simulink model "Processo"  (R2021b)
settings: Solver=ode4  StartTime=0.0  StopTime=1000  FixedStep=1e-1  RelTol=1e-3
model workspace (MAT data in the model file):
  plant_dist = [0  3  3  3  5  4  8  8  6; 3  0  3  3  5  5  8  6  4; 3  3  0  1  3  3  8  6  4; 3  3  1  0  3  3  8  6  4; 5  5  3  3  0  3  6  4  2; 4  5  3  3  3  0  6  6  4; 8  8  8  8  6  6  0  3  5; 8  6  6  6  4  6  3  0  3; 6  4  4  4  2  4  5  3  0]
undefined symbols (not defined in the file): entity, getAttribute, m, n
libraries: simulink x2, sldelib x1
settings Model: PauseTimes=0  Creator=chrez  LastModifiedBy=chrez

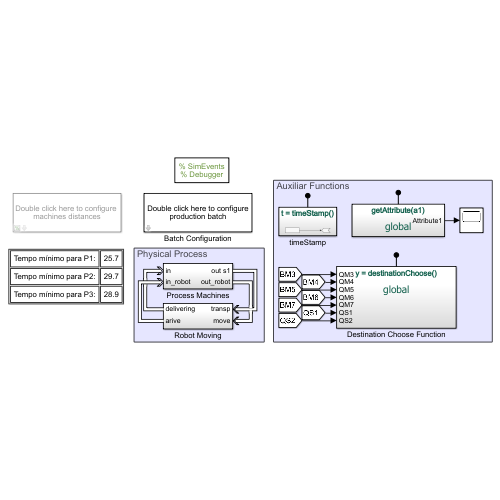
[thumbnail: Simulink's stored preview of the top-level diagram]
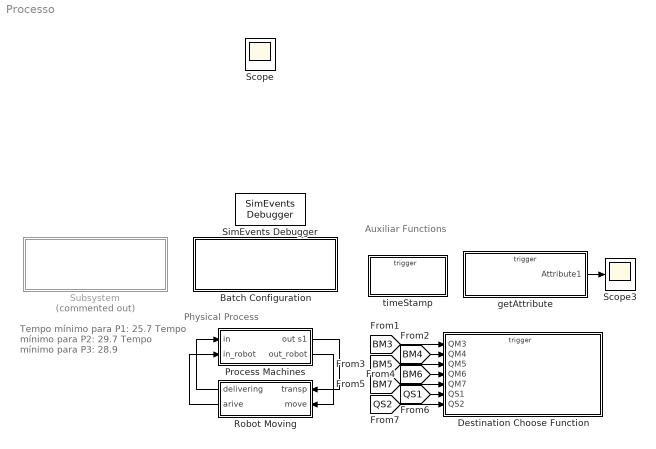
== system Processo ==
  note: Physical Process
  note: Auxiliar Functions
  note: Tempo mínimo para P1:
      | 25.7
      |
      | Tempo mínimo para P2:
      | 29.7
      |
      | Tempo mínimo para P3:
      | 28.9
  Batch Configuration : Subsystem  mask(Batch Configuration){bp1=9, bp2=5, bp3=7, t1recipe=[1 3 4 5 8], t1serviceTimes=[5 3.8 2.5 1.9 1.5], t2recipe=[1 3 6 7 8], t2serviceTimes=[5 3.2 2.4 1.6 2.5], t3recipe=[2 4 5 7 8], t3serviceTimes=[4 2.5 2.4 2.5 2.5]}
      mask prompts: bp1 "Type 1:"; bp2 "Type 2:"; bp3 "Type 3:"; t1recipe "Recipe:"; t1serviceTimes "Service Times:"; t2recipe "Recipe:"; t2serviceTimes "Service Times:"; t3recipe "Recipe:"; t3serviceTimes "Service Times:"
      mask init:
      | assignin('base','bp1',bp1);
      | assignin('base','bp2',bp2);
      | assignin('base','bp3',bp3);
      | assignin('base','t1recipe',t1recipe);
      | assignin('base','t2recipe',t2recipe);
      | assignin('base','t3recipe',t3recipe);
      | assignin('base','t1serviceTimes',t1serviceTimes);
      | assignin('base','t2serviceTimes',t2serviceTimes);
      | assignin('base','t3serviceTimes',t3serviceTimes);
      mask DialogControl ParameterGroupVar Prompt: Batch Query
      mask DialogControl Container7 Prompt: Parts Configuration
      mask DialogControl Container5 Prompt: Type 1
      mask DialogControl Container6 Prompt: Type 2
      mask DialogControl Container10 Prompt: Type 3
      mask Display: disp('Double click here to configure\nproduction batch')
  Destination Choose Function : Subsystem  TreatAsAtomicUnit=on
  Process Machines : Subsystem
  Robot Moving : Subsystem
      settings: PortSchema="{\"entries\":[{\"content\":{\"sides\":[{\"content\":{\"connectorIds\":[\"Out1\",\"Out2\"]},\"type\":\"ConnectorPlacement.EquallySpacedRectSide\",\"uuid\":\"7e07b981-1494-4663-ac57-34fb851c4f8b\"},{\"content\":{\"connectorIds\":[\"In1\",\"In2\"],\"side\":\"RIGHT\"},\"type\":\"ConnectorPlacement.EquallySpacedRectSide\",\"uuid\":\"835ab307-364b-4a91-b206-e24ceecefc82\"},{\"content\":{\"connectorIds\":[],\"side\":\"TOP\"},\"type\":\"ConnectorPlacement.EquallySpacedRectSide\",\"uuid\":\"da88ac6b-0800-49ec-b50d-c8d35a849956\"}]},\"type\":\"ConnectorPlacement.EquallySpacedConnector\",\"uuid\":\"81c2c33b-7057-4473-b38a-1a0a1e572193\"}],\"packageUris\":[\"http://schema.mathworks.com/mf0/Connector/R2020b\"],\"version\":\"1.0\"}"
  Scope3 : Scope
  SimEvents Debugger : sldelib/SimEvents Debugger  EnableDebugger=off  ShowInLibBrowser=0
      settings: SourceProductBaseCode=SE
  Subsystem : Subsystem  Commented=on  mask{m1_2=0, m1_2_copy=0, m1_2_copy_copy=0, m1_2_copy_copy_copy=0, m1_2_copy_copy_copy_copy=0, m1_2_copy_copy_copy_copy_copy=0, m1_2_copy_copy_copy_copy_copy_copy=0, m1_2_copy_copy_copy_copy_copy_copy_copy=0}
      mask prompts: m1_2 "1 - 2"; m1_2_copy "1 - 3"; m1_2_copy_copy "1 - 4"; m1_2_copy_copy_copy "1 - 5"; m1_2_copy_copy_copy_copy "1 - 6"; m1_2_copy_copy_copy_copy_copy "1 - 7"; m1_2_copy_copy_copy_copy_copy_copy "1 - 8"; m1_2_copy_copy_copy_copy_copy_copy_copy "1 - 9"
      mask DialogControl Container3 Prompt: Distances
      mask Display: disp('Double click here to configure \nmachines distances')
  getAttribute : Subsystem  TreatAsAtomicUnit=on
  timeStamp : Subsystem  TreatAsAtomicUnit=on
  Scope : Scope
  wires:
  Process Machines/1(out s1) -> Robot Moving/1(transp)
  Robot Moving/1(delivering) -> Process Machines/1(in)
  Process Machines/2(out_robot) -> Robot Moving/2(move)
  Robot Moving/2(arive) -> Process Machines/2(in_robot)
  [BM3] -> Destination Choose Function/1(QM3)
  [BM4] -> Destination Choose Function/2(QM4)
  [BM5] -> Destination Choose Function/3(QM5)
  [BM6] -> Destination Choose Function/4(QM6)
  [BM7] -> Destination Choose Function/5(QM7)
  getAttribute/1(Attribute1) -> Scope3/1
  [QS1] -> Destination Choose Function/6(QS1)
  [QS2] -> Destination Choose Function/7(QS2)

== system Processo/Batch Configuration ==

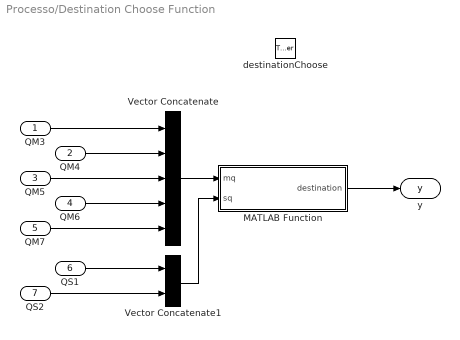
== system Processo/Destination Choose Function ==
  QM3 : Inport
  QM4 : Inport  Port=2
  QM5 : Inport  Port=3
  QM6 : Inport  Port=4
  QM7 : Inport  Port=5
  QS1 : Inport  Port=6
  QS2 : Inport  Port=7
  destinationChoose : TriggerPort  TriggerType=function-call  IsSimulinkFunction=on  FunctionName=destinationChoose  VariantControl=(inherit)
  MATLAB Function : MATLAB Function  TreatAsAtomicUnit=on
  Vector Concatenate : Concatenate  NumInputs=5
  Vector Concatenate1 : Concatenate
  y : ArgOut  DisableCoverage=on  ArgumentName=y
  wires:
  MATLAB Function/1(destination) -> y/1
  QM3/1 -> Vector Concatenate/1
  Vector Concatenate/1 -> MATLAB Function/1(mq)
  QM4/1 -> Vector Concatenate/2
  QM5/1 -> Vector Concatenate/3
  QM6/1 -> Vector Concatenate/4
  QM7/1 -> Vector Concatenate/5
  Vector Concatenate1/1 -> MATLAB Function/2(sq)
  QS2/1 -> Vector Concatenate1/2
  QS1/1 -> Vector Concatenate1/1

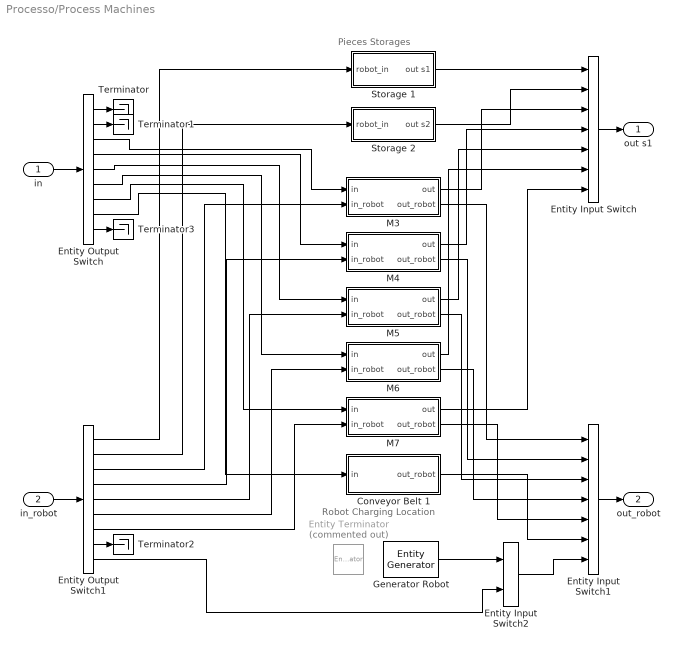
== system Processo/Process Machines ==
  note: Robot Charging Location
  note: Pieces Storages
  in : Inport
  in_robot : Inport  Port=2
  Conveyor Belt 1 : Subsystem
  Entity Input Switch : EntityInputSwitch  InputPortMessageModes=m,m,m,m,m,m,m  OutputPortMessageModes=m  NumberInputPorts=7
      settings: InputPortMap=u1,u2,u3,u4,u5,u6,u7
  Entity Input Switch1 : EntityInputSwitch  InputPortMessageModes=m,m,m,m,m,m,m  OutputPortMessageModes=m  NumberInputPorts=7
      settings: InputPortMap=u1,u2,u3,u4,u5,u6,u7
  Entity Input Switch2 : EntityInputSwitch  InputPortMessageModes=m,m  OutputPortMessageModes=m
  Entity Output Switch : EntityOutputSwitch  InputPortMessageModes=m  OutputPortMessageModes=m,m,m,m,m,m,m,m,m  NumberOutputPorts=9  SwitchingCriterion=From attribute  SwitchAttributeName=robot.atPlace
      settings: OutputPortMap=o0,o1,o2,o3,o4,o5,o6,o7,o8
  Entity Output Switch1 : EntityOutputSwitch  InputPortMessageModes=m  OutputPortMessageModes=m,m,m,m,m,m,m,m,m  NumberOutputPorts=9  SwitchingCriterion=From attribute  SwitchAttributeName=atPlace
      settings: OutputPortMap=o0,o1,o2,o3,o4,o5,o6,o7,o8
  Entity Terminator : EntityTerminator  Commented=on  InputPortMessageModes=m
  Generator Robot : EntityGenerator  OutputPortMessageModes=m  TimeSource=MATLAB action  IntergenerationTimeAction=|  GenerateEntityAtSimulationStart=off  GenerateAction=|  AttributeName=isMoving|atPlace|load|destination  AttributeInitialValue=false|9|0|0  EntityType=Structured  EntityTypeName=robot
      IntergenerationTimeAction=|
      | T = 0;   % fixed intergeneration time
      | N = 1;   % number of entities generated
      | persistent nr;
      | if isempty(nr)
      |   nr = 1;
      | end
      | 
      | if nr <= N
      |   dt = T;
      | else
      |   dt = inf;
      | end
      | nr = nr + 1;
      GenerateAction=|
      | %if rand(1) > 0.5
      | %    robot.destination = 1
      | %else
      | %    robot.destination = 2
      | %end
  M3 : Subsystem
  M4 : Subsystem
  M5 : Subsystem
  M6 : Subsystem
  M7 : Subsystem
  Storage 1 : Subsystem
  Storage 2 : Subsystem
  Terminator{,1..3} (4 alike) : Terminator
  out s1 : Outport
  out_robot : Outport  Port=2
  wires:
  Entity Input Switch/1 -> out s1/1
  Entity Input Switch1/1 -> out_robot/1
  Generator Robot/1 -> Entity Input Switch2/1
  Storage 1/1(out s1) -> Entity Input Switch/1
  in_robot/1 -> Entity Output Switch1/1
  in/1 -> Entity Output Switch/1
  M3/2(out_robot) -> Entity Input Switch1/1
  Entity Output Switch1/9 -> Entity Input Switch2/2
  Entity Output Switch1/1 -> Storage 1/1(robot_in)
  Entity Output Switch1/2 -> Storage 2/1(robot_in)
  Entity Output Switch1/3 -> M3/2(in_robot)
  Entity Output Switch/3 -> M3/1(in)
  Storage 2/1(out s2) -> Entity Input Switch/2
  M3/1(out) -> Entity Input Switch/3
  Entity Output Switch/4 -> M4/1(in)
  Entity Output Switch1/4 -> M4/2(in_robot)
  M4/1(out) -> Entity Input Switch/4
  M4/2(out_robot) -> Entity Input Switch1/2
  Entity Output Switch1/5 -> M5/2(in_robot)
  Entity Output Switch1/6 -> M6/2(in_robot)
  Entity Output Switch1/7 -> M7/2(in_robot)
  Entity Output Switch/5 -> M5/1(in)
  Entity Output Switch/6 -> M6/1(in)
  Entity Output Switch/7 -> M7/1(in)
  M5/1(out) -> Entity Input Switch/5
  M6/1(out) -> Entity Input Switch/6
  M7/1(out) -> Entity Input Switch/7
  M5/2(out_robot) -> Entity Input Switch1/3
  M6/2(out_robot) -> Entity Input Switch1/4
  M7/2(out_robot) -> Entity Input Switch1/5
  Conveyor Belt 1/1(out_robot) -> Entity Input Switch1/6
  Entity Output Switch/8 -> Conveyor Belt 1/1(in)
  Entity Output Switch/1 -> Terminator/1
  Entity Output Switch/2 -> Terminator1/1
  Entity Output Switch1/8 -> Terminator2/1
  Entity Input Switch2/1 -> Entity Input Switch1/7
  Entity Output Switch/9 -> Terminator3/1

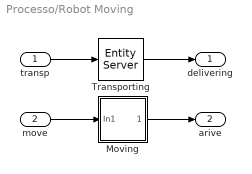
== system Processo/Robot Moving ==
  transp : Inport
  move : Inport  Port=2
  Moving : Subsystem
  Transporting : EntityServer  InputPortMessageModes=m  OutputPortMessageModes=m  Capacity=1  ServiceTimeSource=MATLAB action  ServiceTimeAction=dt = plant_dist(entity.robot.atPlace,entity.robot.destination);  EntryAction=entity.robot.isMoving = true;  ServiceCompleteAction=|
      | entity.robot.atPlace = entity.robot.destination;
      | entity.robot.isMoving = false;
  delivering : Outport
  arive : Outport  Port=2
  wires:
  transp/1 -> Transporting/1
  Transporting/1 -> delivering/1
  move/1 -> Moving/1(In1)
  Moving/1(Out1) -> arive/1

== system Processo/Subsystem ==

== system Processo/getAttribute ==
  getAttribute : TriggerPort  TriggerType=function-call  IsSimulinkFunction=on  FunctionName=getAttribute  VariantControl=Variant
  a1 : ArgIn  ArgumentName=a1
  Attribute1 : Outport  VectorParamsAs1DForOutWhenUnconnected=off
  wires:
  a1/1 -> Attribute1/1

== system Processo/timeStamp ==
  timeStamp : TriggerPort  TriggerType=function-call  IsSimulinkFunction=on  FunctionName=timeStamp  FunctionVisibility=scoped  VariantControl=(inherit)
  Digital Clock : DigitalClock  SampleTime=-1
  t : ArgOut  DisableCoverage=on  ArgumentName=t
  wires:
  Digital Clock/1 -> t/1

== system Processo/Process Machines/Conveyor Belt 1 ==
  in : Inport
  Composite Entity Splitter : CompositeEntitySplitter  InputPortMessageModes=m  OutputPortMessageModes=m,m
      settings: OutputPortMap=o0,o1
  Entity Terminator : EntityTerminator  InputPortMessageModes=m  EntryAction=getAttribute(entity.totalProductionTime);
  Unloading : EntityServer  InputPortMessageModes=m  OutputPortMessageModes=m  Capacity=1  ServiceTimeSource=MATLAB action  ServiceTimeAction=|  ServiceCompleteAction=|
      ServiceTimeAction=|
      | dt = 0;
      | p = 1;
      | for i = entity.part.recipe
      |     if i == 8
      |         dt = entity.part.servicesTimes(p);
      |     end
      |     p = p + 1;
      | end
      ServiceCompleteAction=|
      | entity.part.terminateTimeStamp = timeStamp();
      | 
      | entity.part.totalProductionTime = entity.part.terminateTimeStamp - entity.part.generateTimeStamp;
  out_robot : Outport
  wires:
  in/1 -> Unloading/1
  Unloading/1 -> Composite Entity Splitter/1
  Composite Entity Splitter/1 -> Entity Terminator/1
  Composite Entity Splitter/2 -> out_robot/1

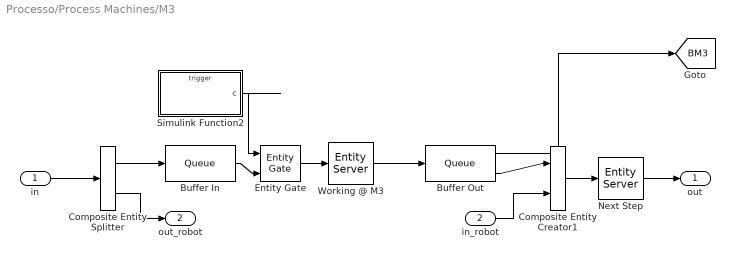
== system Processo/Process Machines/M3 ==
  in : Inport
  in_robot : Inport  Port=2
  Buffer In : Queue  InputPortMessageModes=m  OutputPortMessageModes=m  Capacity=1
  Buffer Out : Queue  InputPortMessageModes=m  OutputPortMessageModes=n,m  Capacity=1  EntryAction=|  ExitAction=|  NumberEntitiesInBlock=on
      EntryAction=|
      | %open = 1;
      | close = 0;
      | GateCtrl(close);
      ExitAction=|
      | open = 1;
      | %close = 0;
      | GateCtrl(open);
      settings: OutputPortMap=o1,o5
  Composite Entity Creator1 : CompositeEntityCreator  InputPortMessageModes=m,m  OutputPortMessageModes=m  EntityTypeName=loaded_robot  InputEntityName=part|robot
      settings: InputPortMap=u0,u1
  Composite Entity Splitter : CompositeEntitySplitter  InputPortMessageModes=m  OutputPortMessageModes=m,m
      settings: OutputPortMap=o0,o1
  Entity Gate : EntityGate  InputPortMessageModes=m,m  OutputPortMessageModes=m  OpenGateAtSimulationStart=on
  Next Step : EntityServer  InputPortMessageModes=m  OutputPortMessageModes=m  Capacity=1  ServiceTimeValue=0  ServiceCompleteAction=|
      | p = 1;
      | for i = entity.part.recipe
      |     if i == 3
      |         entity.robot.destination = entity.part.recipe(p+1);
      |         break
      |     end
      |     p = p + 1;
      | end
      | 
      | %entity.robot.destination = find(entity.part.recipe==3)+1
  Simulink Function2 : Subsystem  TreatAsAtomicUnit=on
  Working @ M3 : EntityServer  InputPortMessageModes=m  OutputPortMessageModes=m  Capacity=1  ServiceTimeSource=MATLAB action  ServiceTimeValue=38  ServiceTimeAttributeName=serviceTime  ServiceTimeAction=|
      | dt = 0;
      | p = 1;
      | for i = entity.recipe
      |     if i == 3
      |         dt = entity.servicesTimes(p);
      |         break
      |     end
      |     p = p + 1;
      | end
  out : Outport
  out_robot : Outport  Port=2
  tag scope: BM3=global
  wires:
  Buffer In/1 -> Entity Gate/2
  Working @ M3/1 -> Buffer Out/1
  Composite Entity Splitter/1 -> Buffer In/1
  Buffer Out/2 -> Composite Entity Creator1/1
  in_robot/1 -> Composite Entity Creator1/2
  Composite Entity Splitter/2 -> out_robot/1
  in/1 -> Composite Entity Splitter/1
  Composite Entity Creator1/1 -> Next Step/1
  Next Step/1 -> out/1
  Entity Gate/1 -> Working @ M3/1
  Buffer Out/1 -> [BM3]
  Simulink Function2/1(c) -> Entity Gate/1

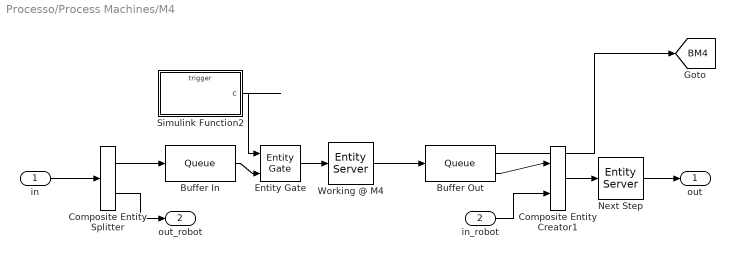
== system Processo/Process Machines/M4 ==
  in : Inport
  in_robot : Inport  Port=2
  Buffer In : Queue  InputPortMessageModes=m  OutputPortMessageModes=m  Capacity=1
  Buffer Out : Queue  InputPortMessageModes=m  OutputPortMessageModes=n,m  Capacity=1  EntryAction=|  ExitAction=|  NumberEntitiesInBlock=on
      EntryAction=|
      | %open = 1;
      | close = 0;
      | GateCtrl(close);
      ExitAction=|
      | open = 1;
      | %close = 0;
      | GateCtrl(open);
      settings: OutputPortMap=o1,o5
  Composite Entity Creator1 : CompositeEntityCreator  InputPortMessageModes=m,m  OutputPortMessageModes=m  EntityTypeName=loaded_robot  InputEntityName=part|robot
      settings: InputPortMap=u0,u1
  Composite Entity Splitter : CompositeEntitySplitter  InputPortMessageModes=m  OutputPortMessageModes=m,m
      settings: OutputPortMap=o0,o1
  Entity Gate : EntityGate  InputPortMessageModes=m,m  OutputPortMessageModes=m  OpenGateAtSimulationStart=on
  Next Step : EntityServer  InputPortMessageModes=m  OutputPortMessageModes=m  Capacity=1  ServiceTimeValue=0  ServiceCompleteAction=|
      | p = 1;
      | for i = entity.part.recipe
      |     if i == 4
      |         entity.robot.destination = entity.part.recipe(p+1);
      |         break
      |     end
      |     p = p + 1;
      | end
      | 
      | %entity.robot.destination = find(entity.part.recipe==3)+1
  Simulink Function2 : Subsystem  TreatAsAtomicUnit=on
  Working @ M4 : EntityServer  InputPortMessageModes=m  OutputPortMessageModes=m  Capacity=1  ServiceTimeSource=MATLAB action  ServiceTimeValue=38  ServiceTimeAttributeName=serviceTime  ServiceTimeAction=|
      | dt = 0;
      | p = 1;
      | for i = entity.recipe
      |     if i == 4
      |         dt = entity.servicesTimes(p);
      |         break
      |     end
      |     p = p + 1;
      | end
  out : Outport
  out_robot : Outport  Port=2
  tag scope: BM4=global
  wires:
  Buffer In/1 -> Entity Gate/2
  Working @ M4/1 -> Buffer Out/1
  Composite Entity Splitter/1 -> Buffer In/1
  Buffer Out/2 -> Composite Entity Creator1/1
  in_robot/1 -> Composite Entity Creator1/2
  Composite Entity Splitter/2 -> out_robot/1
  in/1 -> Composite Entity Splitter/1
  Composite Entity Creator1/1 -> Next Step/1
  Next Step/1 -> out/1
  Entity Gate/1 -> Working @ M4/1
  Buffer Out/1 -> [BM4]
  Simulink Function2/1(c) -> Entity Gate/1

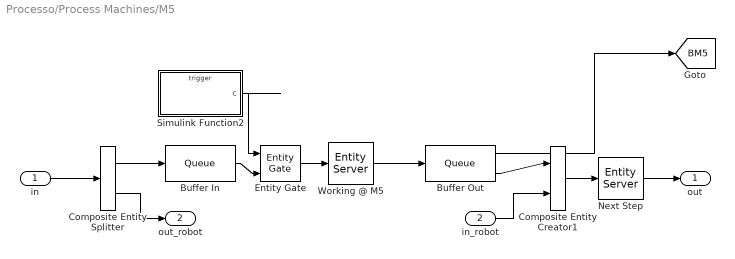
== system Processo/Process Machines/M5 ==
  in : Inport
  in_robot : Inport  Port=2
  Buffer In : Queue  InputPortMessageModes=m  OutputPortMessageModes=m  Capacity=1
  Buffer Out : Queue  InputPortMessageModes=m  OutputPortMessageModes=n,m  Capacity=1  EntryAction=|  ExitAction=|  NumberEntitiesInBlock=on
      EntryAction=|
      | %open = 1;
      | close = 0;
      | GateCtrl(close);
      ExitAction=|
      | open = 1;
      | %close = 0;
      | GateCtrl(open);
      settings: OutputPortMap=o1,o5
  Composite Entity Creator1 : CompositeEntityCreator  InputPortMessageModes=m,m  OutputPortMessageModes=m  EntityTypeName=loaded_robot  InputEntityName=part|robot
      settings: InputPortMap=u0,u1
  Composite Entity Splitter : CompositeEntitySplitter  InputPortMessageModes=m  OutputPortMessageModes=m,m
      settings: OutputPortMap=o0,o1
  Entity Gate : EntityGate  InputPortMessageModes=m,m  OutputPortMessageModes=m  OpenGateAtSimulationStart=on
  Next Step : EntityServer  InputPortMessageModes=m  OutputPortMessageModes=m  Capacity=1  ServiceTimeValue=0  ServiceCompleteAction=|
      | p = 1;
      | for i = entity.part.recipe
      |     if i == 5
      |         entity.robot.destination = entity.part.recipe(p+1);
      |         break
      |     end
      |     p = p + 1;
      | end
      | 
      | %entity.robot.destination = find(entity.part.recipe==3)+1
  Simulink Function2 : Subsystem  TreatAsAtomicUnit=on
  Working @ M5 : EntityServer  InputPortMessageModes=m  OutputPortMessageModes=m  Capacity=1  ServiceTimeSource=MATLAB action  ServiceTimeValue=38  ServiceTimeAttributeName=serviceTime  ServiceTimeAction=|
      | dt = 0;
      | p = 1;
      | for i = entity.recipe
      |     if i == 5
      |         dt = entity.servicesTimes(p);
      |         break
      |     end
      |     p = p + 1;
      | end
  out : Outport
  out_robot : Outport  Port=2
  tag scope: BM5=global
  wires:
  Buffer In/1 -> Entity Gate/2
  Working @ M5/1 -> Buffer Out/1
  Composite Entity Splitter/1 -> Buffer In/1
  Buffer Out/2 -> Composite Entity Creator1/1
  in_robot/1 -> Composite Entity Creator1/2
  Composite Entity Splitter/2 -> out_robot/1
  in/1 -> Composite Entity Splitter/1
  Composite Entity Creator1/1 -> Next Step/1
  Next Step/1 -> out/1
  Entity Gate/1 -> Working @ M5/1
  Buffer Out/1 -> [BM5]
  Simulink Function2/1(c) -> Entity Gate/1

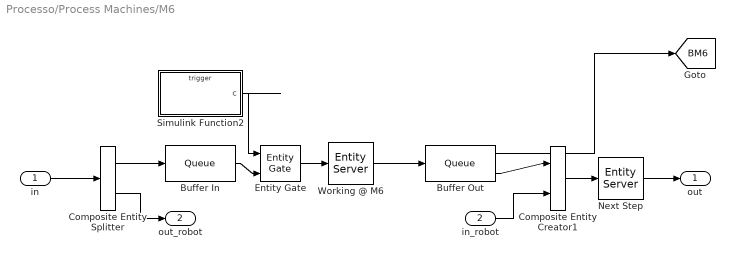
== system Processo/Process Machines/M6 ==
  in : Inport
  in_robot : Inport  Port=2
  Buffer In : Queue  InputPortMessageModes=m  OutputPortMessageModes=m  Capacity=1
  Buffer Out : Queue  InputPortMessageModes=m  OutputPortMessageModes=n,m  Capacity=1  EntryAction=|  ExitAction=|  NumberEntitiesInBlock=on
      EntryAction=|
      | %open = 1;
      | close = 0;
      | GateCtrl(close);
      ExitAction=|
      | open = 1;
      | %close = 0;
      | GateCtrl(open);
      settings: OutputPortMap=o1,o5
  Composite Entity Creator1 : CompositeEntityCreator  InputPortMessageModes=m,m  OutputPortMessageModes=m  EntityTypeName=loaded_robot  InputEntityName=part|robot
      settings: InputPortMap=u0,u1
  Composite Entity Splitter : CompositeEntitySplitter  InputPortMessageModes=m  OutputPortMessageModes=m,m
      settings: OutputPortMap=o0,o1
  Entity Gate : EntityGate  InputPortMessageModes=m,m  OutputPortMessageModes=m  OpenGateAtSimulationStart=on
  Next Step : EntityServer  InputPortMessageModes=m  OutputPortMessageModes=m  Capacity=1  ServiceTimeValue=0  ServiceCompleteAction=|
      | p = 1;
      | for i = entity.part.recipe
      |     if i == 6
      |         entity.robot.destination = entity.part.recipe(p+1);
      |         break
      |     end
      |     p = p + 1;
      | end
      | 
      | %entity.robot.destination = find(entity.part.recipe==3)+1
  Simulink Function2 : Subsystem  TreatAsAtomicUnit=on
  Working @ M6 : EntityServer  InputPortMessageModes=m  OutputPortMessageModes=m  Capacity=1  ServiceTimeSource=MATLAB action  ServiceTimeValue=38  ServiceTimeAttributeName=serviceTime  ServiceTimeAction=|
      | dt = 0;
      | p = 1;
      | for i = entity.recipe
      |     if i == 6
      |         dt = entity.servicesTimes(p);
      |         break
      |     end
      |     p = p + 1;
      | end
  out : Outport
  out_robot : Outport  Port=2
  tag scope: BM6=global
  wires:
  Buffer In/1 -> Entity Gate/2
  Working @ M6/1 -> Buffer Out/1
  Composite Entity Splitter/1 -> Buffer In/1
  Buffer Out/2 -> Composite Entity Creator1/1
  in_robot/1 -> Composite Entity Creator1/2
  Composite Entity Splitter/2 -> out_robot/1
  in/1 -> Composite Entity Splitter/1
  Composite Entity Creator1/1 -> Next Step/1
  Next Step/1 -> out/1
  Entity Gate/1 -> Working @ M6/1
  Buffer Out/1 -> [BM6]
  Simulink Function2/1(c) -> Entity Gate/1

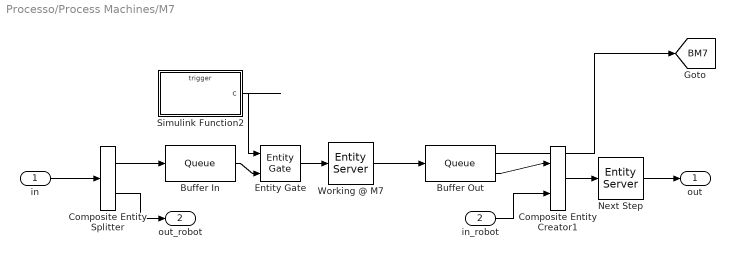
== system Processo/Process Machines/M7 ==
  in : Inport
  in_robot : Inport  Port=2
  Buffer In : Queue  InputPortMessageModes=m  OutputPortMessageModes=m  Capacity=1
  Buffer Out : Queue  InputPortMessageModes=m  OutputPortMessageModes=n,m  Capacity=1  EntryAction=|  ExitAction=|  NumberEntitiesInBlock=on
      EntryAction=|
      | %open = 1;
      | close = 0;
      | GateCtrl(close);
      ExitAction=|
      | open = 1;
      | %close = 0;
      | GateCtrl(open);
      settings: OutputPortMap=o1,o5
  Composite Entity Creator1 : CompositeEntityCreator  InputPortMessageModes=m,m  OutputPortMessageModes=m  EntityTypeName=loaded_robot  InputEntityName=part|robot
      settings: InputPortMap=u0,u1
  Composite Entity Splitter : CompositeEntitySplitter  InputPortMessageModes=m  OutputPortMessageModes=m,m
      settings: OutputPortMap=o0,o1
  Entity Gate : EntityGate  InputPortMessageModes=m,m  OutputPortMessageModes=m  OpenGateAtSimulationStart=on
  Next Step : EntityServer  InputPortMessageModes=m  OutputPortMessageModes=m  Capacity=1  ServiceTimeValue=0  ServiceCompleteAction=|
      | p = 1;
      | for i = entity.part.recipe
      |     if i == 7
      |         entity.robot.destination = entity.part.recipe(p+1);
      |         break
      |     end
      |     p = p + 1;
      | end
      | 
      | %entity.robot.destination = find(entity.part.recipe==3)+1
  Simulink Function2 : Subsystem  TreatAsAtomicUnit=on
  Working @ M7 : EntityServer  InputPortMessageModes=m  OutputPortMessageModes=m  Capacity=1  ServiceTimeSource=MATLAB action  ServiceTimeValue=38  ServiceTimeAttributeName=serviceTime  ServiceTimeAction=|
      | dt = 0;
      | p = 1;
      | for i = entity.recipe
      |     if i == 7
      |         dt = entity.servicesTimes(p);
      |         break
      |     end
      |     p = p + 1;
      | end
  out : Outport
  out_robot : Outport  Port=2
  tag scope: BM7=global
  wires:
  Buffer In/1 -> Entity Gate/2
  Working @ M7/1 -> Buffer Out/1
  Composite Entity Splitter/1 -> Buffer In/1
  Buffer Out/2 -> Composite Entity Creator1/1
  in_robot/1 -> Composite Entity Creator1/2
  Composite Entity Splitter/2 -> out_robot/1
  in/1 -> Composite Entity Splitter/1
  Composite Entity Creator1/1 -> Next Step/1
  Next Step/1 -> out/1
  Entity Gate/1 -> Working @ M7/1
  Buffer Out/1 -> [BM7]
  Simulink Function2/1(c) -> Entity Gate/1

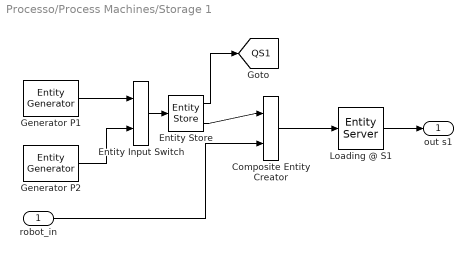
== system Processo/Process Machines/Storage 1 ==
  robot_in : Inport
  Composite Entity Creator : CompositeEntityCreator  InputPortMessageModes=m,m  OutputPortMessageModes=m  EntityTypeName=loaded_robot  InputEntityName=part|robot
      settings: InputPortMap=u0,u1
  Entity Input Switch : EntityInputSwitch  InputPortMessageModes=m,m  OutputPortMessageModes=m
  Entity Store : EntityStore  InputPortMessageModes=m  OutputPortMessageModes=n,m  Capacity=Inf  NumberEntitiesInBlock=on
      settings: OutputPortMap=o1,o4
  Generator P1 : EntityGenerator  OutputPortMessageModes=m  TimeSource=MATLAB action  IntergenerationTimeAction=|  GenerateEntityAtSimulationStart=off  GenerateAction=|  AttributeName=type|recipe|servicesTimes|generateTimeStamp|terminateTimeStamp|totalProductionTime  AttributeInitialValue=1|[0 0 0 0 0]|[0 0 0 0 0]|0|0|0  EntityType=Structured  EntityTypeName=part
      IntergenerationTimeAction=|
      | T = 0;   % fixed intergeneration time
      | N = bp1;   % number of entities generated
      | persistent nr;
      | if isempty(nr)
      |   nr = 1;
      | end
      | 
      | if nr <= N
      |   dt = T;
      | else
      |   dt = inf;
      | end
      | nr = nr + 1;
      GenerateAction=|
      | entity.recipe = t1recipe;
      | entity.servicesTimes = t1serviceTimes;
  Generator P2 : EntityGenerator  OutputPortMessageModes=m  TimeSource=MATLAB action  IntergenerationTimeAction=|  GenerateEntityAtSimulationStart=off  GenerateAction=|  AttributeName=type|recipe|servicesTimes|generateTimeStamp|terminateTimeStamp|totalProductionTime  AttributeInitialValue=2|[0 0 0 0 0]|[0 0 0 0 0]|0|0|0  EntityType=Structured  EntityTypeName=part
      IntergenerationTimeAction=|
      | T = 0;   % fixed intergeneration time
      | N = bp2;   % number of entities generated
      | persistent nr;
      | if isempty(nr)
      |   nr = 1;
      | end
      | 
      | if nr <= N
      |   dt = T;
      | else
      |   dt = inf;
      | end
      | nr = nr + 1;
      GenerateAction=|
      | entity.recipe = t2recipe;
      | entity.servicesTimes = t2serviceTimes;
  Loading @ S1 : EntityServer  InputPortMessageModes=m  OutputPortMessageModes=m  Capacity=1  ServiceTimeSource=MATLAB action  ServiceTimeValue=5  ServiceTimeAction=|  EntryAction=entity.part.generateTimeStamp = timeStamp();  ServiceCompleteAction=|
      ServiceTimeAction=|
      | dt = 0;
      | p = 1;
      | for i = entity.part.recipe
      |     if i == 1
      |         dt = entity.part.servicesTimes(p);
      |         break
      |     end
      |     p = p + 1;
      | end
      ServiceCompleteAction=|
      | p = 1;
      | for i = entity.part.recipe
      |     if i == 1
      |         entity.robot.destination = entity.part.recipe(p+1);
      |         break
      |     end
      |     p = p + 1;
      | end
  out s1 : Outport
  tag scope: QS1=global
  wires:
  Loading @ S1/1 -> out s1/1
  Entity Input Switch/1 -> Entity Store/1
  Generator P2/1 -> Entity Input Switch/2
  Generator P1/1 -> Entity Input Switch/1
  Composite Entity Creator/1 -> Loading @ S1/1
  Entity Store/2 -> Composite Entity Creator/1
  robot_in/1 -> Composite Entity Creator/2
  Entity Store/1 -> [QS1]

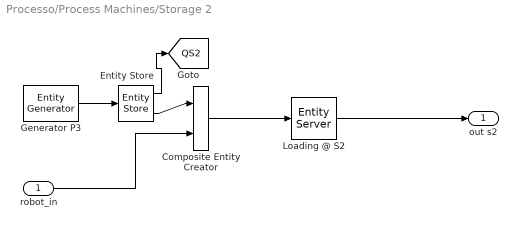
== system Processo/Process Machines/Storage 2 ==
  robot_in : Inport
  Composite Entity Creator : CompositeEntityCreator  InputPortMessageModes=m,m  OutputPortMessageModes=m  EntityTypeName=loaded_robot  InputEntityName=part|robot
      settings: InputPortMap=u0,u1
  Entity Store : EntityStore  InputPortMessageModes=m  OutputPortMessageModes=n,m  Capacity=Inf  NumberEntitiesInBlock=on
      settings: OutputPortMap=o1,o4
  Generator P3 : EntityGenerator  OutputPortMessageModes=m  TimeSource=MATLAB action  IntergenerationTimeAction=|  GenerateEntityAtSimulationStart=off  GenerateAction=|  AttributeName=type|recipe|servicesTimes|generateTimeStamp|terminateTimeStamp|totalProductionTime  AttributeInitialValue=3|[0 0 0 0 0]|[0 0 0 0 0]|0|0|0  EntityType=Structured  EntityTypeName=part
      IntergenerationTimeAction=|
      | T = 0;   % fixed intergeneration time
      | N = bp3;   % number of entities generated
      | persistent nr;
      | if isempty(nr)
      |   nr = 1;
      | end
      | 
      | if nr <= N
      |   dt = T;
      | else
      |   dt = inf;
      | end
      | nr = nr + 1;
      GenerateAction=|
      | entity.recipe = t3recipe;
      | entity.servicesTimes = t3serviceTimes;
  Loading @ S2 : EntityServer  InputPortMessageModes=m  OutputPortMessageModes=m  Capacity=1  ServiceTimeSource=MATLAB action  ServiceTimeValue=4  ServiceTimeAction=|  EntryAction=entity.part.generateTimeStamp = timeStamp();  ServiceCompleteAction=|
      ServiceTimeAction=|
      | dt = 0;
      | for i = entity.part.recipe
      |     if i == 2
      |         dt = entity.part.recipe(i);
      |         break
      |     end
      | end
      ServiceCompleteAction=|
      | p = 1;
      | for i = entity.part.recipe
      |     if i == 2
      |         entity.robot.destination = entity.part.recipe(p+1);
      |         break
      |     end
      |     p = p + 1;
      | end
  out s2 : Outport
  tag scope: QS2=global
  wires:
  Loading @ S2/1 -> out s2/1
  Generator P3/1 -> Entity Store/1
  Composite Entity Creator/1 -> Loading @ S2/1
  Entity Store/2 -> Composite Entity Creator/1
  robot_in/1 -> Composite Entity Creator/2
  Entity Store/1 -> [QS2]

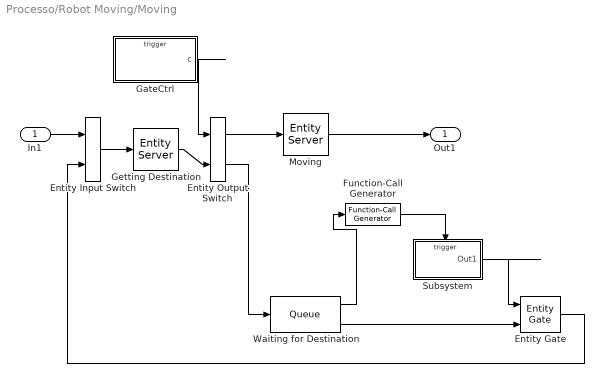
== system Processo/Robot Moving/Moving ==
  In1 : Inport
  Entity Input Switch : EntityInputSwitch  InputPortMessageModes=m,m  OutputPortMessageModes=m
  Entity Output Switch : EntityOutputSwitch  InputPortMessageModes=m,m  OutputPortMessageModes=m,m  SwitchingCriterion=From control port  SwitchAttributeName=Attribute1  InitialPortSelection=2
      settings: InputPortMap=u0,u1
  Entity Gate : EntityGate  InputPortMessageModes=m,m  OutputPortMessageModes=m  OperatingMode=Release gate
  Function-Call Generator : simulink/Ports & Subsystems/Function-Call Generator  sample_time=0.1  numberOfIterations=1  DisallowWideOutput=off  ShowEnablePort=on
  GateCtrl : Subsystem  TreatAsAtomicUnit=on
  Getting Destination : EntityServer  InputPortMessageModes=m  OutputPortMessageModes=m  Capacity=1  ServiceTimeValue=0  ServiceCompleteAction=|
      | close = 2;
      | open = 1;
      | 
      | destination = destinationChoose();
      | if destination == 0
      |     GateCtrl(close); 
      |         % o problema está aqui!
      |         % quando o gate fecha, não tenho uma maneira
      |         % de verificar se pode abrir ele de novo...
      |         %destination = entity.atPlace;
      | else
      |     GateCtrl(open);
      | end
      | entity.destination = destination;
  Moving : EntityServer  InputPortMessageModes=m  OutputPortMessageModes=m  Capacity=1  ServiceTimeSource=MATLAB action  ServiceTimeAction=dt = plant_dist(entity.atPlace,entity.destination);  EntryAction=entity.isMoving = true;  ServiceCompleteAction=|
      | entity.atPlace = entity.destination;
      | entity.isMoving = false;
  Subsystem : Subsystem
  Waiting for Destination : Queue  InputPortMessageModes=m  OutputPortMessageModes=n,m  Capacity=1  NumberEntitiesInBlock=on
      settings: OutputPortMap=o1,o5
  Out1 : Outport
  wires:
  Moving/1 -> Out1/1
  Entity Output Switch/1 -> Moving/1
  Waiting for Destination/2 -> Entity Gate/2
  In1/1 -> Entity Input Switch/1
  GateCtrl/1(c) -> Entity Output Switch/1
  Waiting for Destination/1 -> Function-Call Generator/1
  Getting Destination/1 -> Entity Output Switch/2
  Entity Output Switch/2 -> Waiting for Destination/1
  Entity Input Switch/1 -> Getting Destination/1
  Entity Gate/1 -> Entity Input Switch/2
  Function-Call Generator/1 -> Subsystem/Trigger
  Subsystem/1(Out1) -> Entity Gate/1

== system Processo/Process Machines/M3/Simulink Function2 ==
  GateCtrl : TriggerPort  TriggerType=function-call  IsSimulinkFunction=on  FunctionName=GateCtrl  FunctionVisibility=scoped  VariantControl=Variant
  Message Send : Send  OutputPortMessageModes=m
  cmd : ArgIn  ArgumentName=cmd
  c : Outport  VectorParamsAs1DForOutWhenUnconnected=off
  wires:
  cmd/1 -> Message Send/1
  Message Send/1 -> c/1

== system Processo/Process Machines/M4/Simulink Function2 ==
  GateCtrl : TriggerPort  TriggerType=function-call  IsSimulinkFunction=on  FunctionName=GateCtrl  FunctionVisibility=scoped  VariantControl=Variant
  Message Send : Send  OutputPortMessageModes=m
  cmd : ArgIn  ArgumentName=cmd
  c : Outport  VectorParamsAs1DForOutWhenUnconnected=off
  wires:
  cmd/1 -> Message Send/1
  Message Send/1 -> c/1

== system Processo/Process Machines/M5/Simulink Function2 ==
  GateCtrl : TriggerPort  TriggerType=function-call  IsSimulinkFunction=on  FunctionName=GateCtrl  FunctionVisibility=scoped  VariantControl=Variant
  Message Send : Send  OutputPortMessageModes=m
  cmd : ArgIn  ArgumentName=cmd
  c : Outport  VectorParamsAs1DForOutWhenUnconnected=off
  wires:
  cmd/1 -> Message Send/1
  Message Send/1 -> c/1

== system Processo/Process Machines/M6/Simulink Function2 ==
  GateCtrl : TriggerPort  TriggerType=function-call  IsSimulinkFunction=on  FunctionName=GateCtrl  FunctionVisibility=scoped  VariantControl=Variant
  Message Send : Send  OutputPortMessageModes=m
  cmd : ArgIn  ArgumentName=cmd
  c : Outport  VectorParamsAs1DForOutWhenUnconnected=off
  wires:
  cmd/1 -> Message Send/1
  Message Send/1 -> c/1

== system Processo/Process Machines/M7/Simulink Function2 ==
  GateCtrl : TriggerPort  TriggerType=function-call  IsSimulinkFunction=on  FunctionName=GateCtrl  FunctionVisibility=scoped  VariantControl=Variant
  Message Send : Send  OutputPortMessageModes=m
  cmd : ArgIn  ArgumentName=cmd
  c : Outport  VectorParamsAs1DForOutWhenUnconnected=off
  wires:
  cmd/1 -> Message Send/1
  Message Send/1 -> c/1

== system Processo/Robot Moving/Moving/GateCtrl ==
  GateCtrl : TriggerPort  TriggerType=function-call  IsSimulinkFunction=on  FunctionName=GateCtrl  FunctionVisibility=scoped  VariantControl=Variant
  Message Send : Send  OutputPortMessageModes=m
  cmd : ArgIn  ArgumentName=cmd
  c : Outport  VectorParamsAs1DForOutWhenUnconnected=off
  wires:
  cmd/1 -> Message Send/1
  Message Send/1 -> c/1

== system Processo/Robot Moving/Moving/Subsystem ==
  Trigger : TriggerPort  TriggerType=function-call  VariantControl=(inherit)  PortDimensions=1
  Compare To Zero : simulink/Logic and Bit Operations/Compare To Zero  relop=>  OutDataTypeStr=boolean
  Function Caller : FunctionCaller  FunctionPrototype=y = destinationChoose()  InputArgumentSpecifications=<Enter example>  OutputArgumentSpecifications=<Enter example>
  Message Send : Send  OutputPortMessageModes=m  ShowEnablePort=on
      settings: InputPortMap=e0,u1
  Out1 : Outport
  wires:
  Function Caller/1 -> Compare To Zero/1
  Message Send/1 -> Out1/1
  Compare To Zero/1 -> Message Send/1, Message Send/2

== matlab function Processo/Destination Choose Function/MATLAB Function ==
  data: mq input; destination output; sq input
function destination = fcn(mq,sq)

mq_select = find(mq)+2;
sq_select = find(sq);

chosen = 0;

if ~isempty(mq_select)
    %chosen = randsample(mq_select,1);
    chosen = mq_select(randsample(length(mq_select),1));
    %chosen = datasample(mq_select,1,'Replace',false);
else
    if ~isempty(sq_select)
        %chosen = randsample(sq_select,1);
        chosen = sq_select(randsample(length(sq_select),1));
        %chosen = datasample(sq_select,1,'Replace',false);
    end
end

destination = chosen;
